simulink model "Taller3_TDCM_Galo"  (R2024a)
settings: Solver=VariableStepAuto  StartTime=0.0  StopTime=120  RelTol=1e-3
libraries: opcualib x2, sldrtlib x1
settings Model: Creator=emili  LastModifiedBy=emili

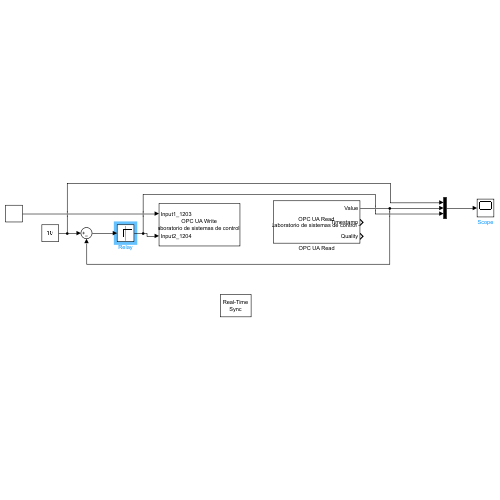
[thumbnail: Simulink's stored preview of the top-level diagram]
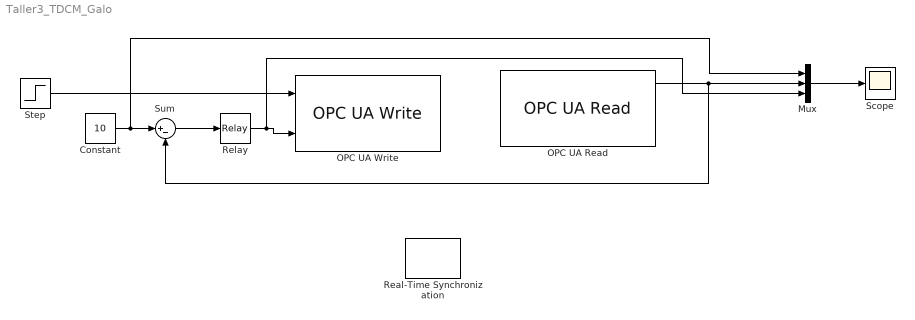
== system Taller3_TDCM_Galo ==
  Constant : Constant  Value=10
  Mux : Mux  Inputs=3
  OPC UA Read : opcualib/OPC UA Read  SelectedServer=UCuenca - Laboratorio de sistemas de control - open62541  ServerList=UCuenca - Laboratorio de sistemas de control - open62541  NodeList={ '1', 'Output', '1', '1205', '1' }  ShowQualityPort=on  ShowTimestampPort=on  ShowTimestampPortAs=Seconds since start  SampleTime=-1
  OPC UA Write : opcualib/OPC UA Write  SelectedServer=UCuenca - Laboratorio de sistemas de control - open62541  ServerList=UCuenca - Laboratorio de sistemas de control - open62541  SampleTime=-1  NodeList={ '1', 'Input1', '1', '1203', '1'; '2', 'Input2', '1', '1204', '1' }
  Real-Time Synchronization : sldrtlib/Real-Time Synchronization  SampleTime=0.2  MaxMissedTicks=10  ShowMissedTicks=off  YieldWhenWaiting=off
  Relay : Relay  OnSwitchValue=0.1  OffSwitchValue=-0.1  OnOutputValue=0  OffOutputValue=1
  Scope : Scope
  Step : Step  After=60  SampleTime=0
  Sum : Sum  Inputs=|+-
  wires:
  OPC UA Read/1 -> Mux/2, Sum/2
  Step/1 -> OPC UA Write/1
  Sum/1 -> Relay/1
  Relay/1 -> Mux/3, OPC UA Write/2
  Mux/1 -> Scope/1
  Constant/1 -> Mux/1, Sum/1
